simulink library "cam"  (Simulink 8.1)
settings: Solver=ode45  StartTime=0.0  StopTime=10.0  RelTol=1e-3
undefined symbols (not defined in the file or in its folder): ENUM_CAMSTATUS_NO_FAILSAFE, ENUM_SENSORSTATE_FAILURE, ENUM_SENSORSTATE_NORMAL, ENUM_SENSORSTATE_NOT_REL
settings Model: Creator=xsellart  LastModifiedBy=tescamilla

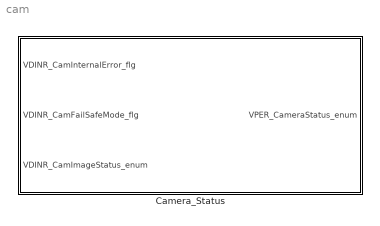
== system cam ==
  Camera_Status : Subsystem

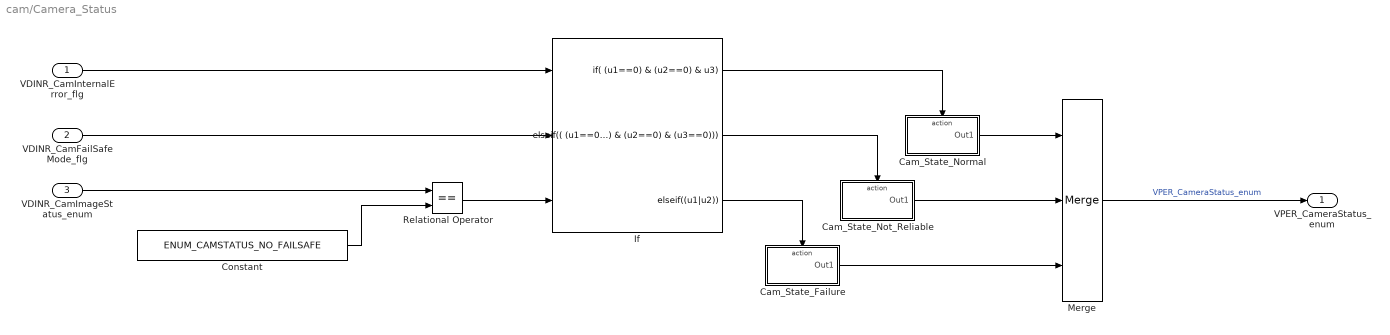
== system cam/Camera_Status ==
  VDINR_CamInternalError_flg : Inport
  VDINR_CamFailSafeMode_flg : Inport  Port=2
  VDINR_CamImageStatus_enum : Inport  Port=3
  Cam_State_Failure : Subsystem  TreatAsAtomicUnit=on
  Cam_State_Normal : Subsystem  TreatAsAtomicUnit=on
  Cam_State_Not_Reliable : Subsystem  TreatAsAtomicUnit=on
  Constant : Constant  Value=ENUM_CAMSTATUS_NO_FAILSAFE
  If : If  NumInputs=3  IfExpression=(u1==0) & (u2==0) & u3  ElseIfExpressions=( (u1==0) & (u2==0) & (u3==0)), (u1|u2)  ShowElse=off
  Merge : Merge  Inputs=3
  Relational Operator : RelationalOperator  Operator===  OutDataTypeStr=boolean
  VPER_CameraStatus_enum : Outport
  wires:
  VDINR_CamImageStatus_enum/1 -> Relational Operator/1
  Cam_State_Not_Reliable/1(Out1) -> Merge/2
  Merge/1 -> VPER_CameraStatus_enum/1  "VPER_CameraStatus_enum"
  Cam_State_Failure/1(Out1) -> Merge/3
  Cam_State_Normal/1(Out1) -> Merge/1
  If/1 -> Cam_State_Normal/Action
  VDINR_CamFailSafeMode_flg/1 -> If/2
  VDINR_CamInternalError_flg/1 -> If/1
  If/3 -> Cam_State_Failure/Action
  Constant/1 -> Relational Operator/2
  Relational Operator/1 -> If/3
  If/2 -> Cam_State_Not_Reliable/Action

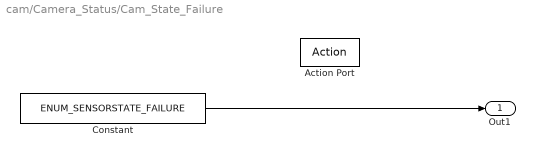
== system cam/Camera_Status/Cam_State_Failure ==
  Action Port : ActionPort  ActionType=elseif
  Constant : Constant  Value=ENUM_SENSORSTATE_FAILURE
  Out1 : Outport
  wires:
  Constant/1 -> Out1/1

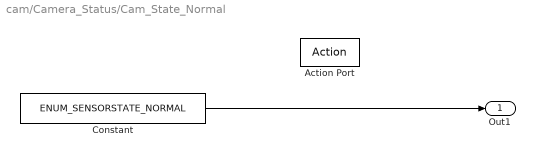
== system cam/Camera_Status/Cam_State_Normal ==
  Action Port : ActionPort  ActionType=then
  Constant : Constant  Value=ENUM_SENSORSTATE_NORMAL
  Out1 : Outport
  wires:
  Constant/1 -> Out1/1

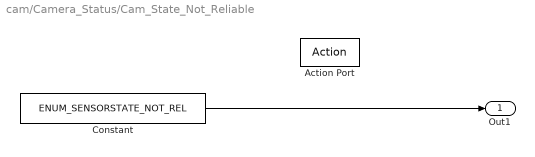
== system cam/Camera_Status/Cam_State_Not_Reliable ==
  Action Port : ActionPort  ActionType=elseif
  Constant : Constant  Value=ENUM_SENSORSTATE_NOT_REL
  Out1 : Outport
  wires:
  Constant/1 -> Out1/1
